simulink model "quat2mat"  (Simulink 6.1)
settings: Solver=ode45  StartTime=0.0  StopTime=10.0  RelTol=1e-3
libraries: simulink x1
settings Model: LastModifiedBy=okawa
settings DebuggingCC: SolverPrmCheckMsg=warning

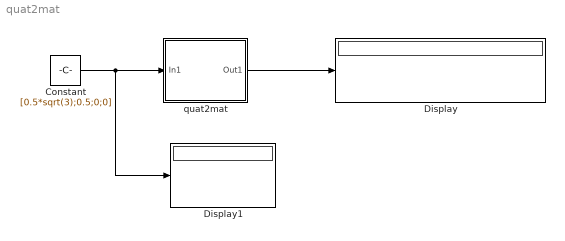
== system quat2mat ==
  Constant : Constant  Value=[0.5*sqrt(3);0.5;0;0]  VectorParams1D=off
  Display : Display
  Display1 : Display
  quat2mat : Subsystem
  wires:
  Constant/1 -> quat2mat/1(In1), Display1/1
  quat2mat/1(Out1) -> Display/1

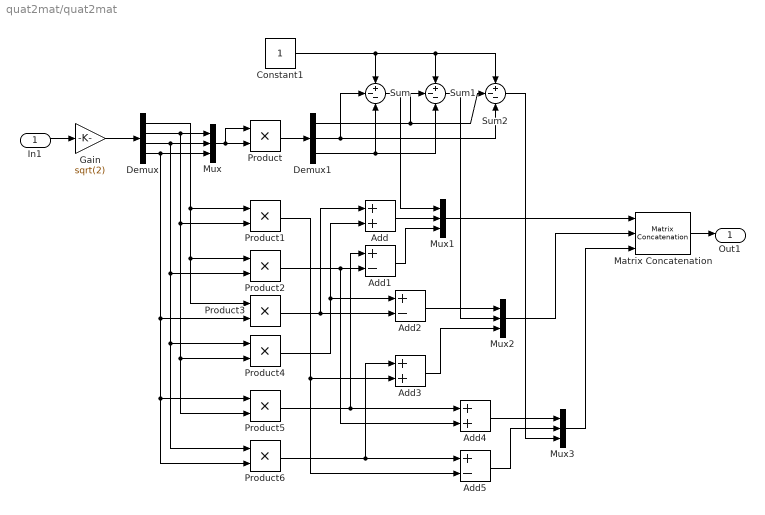
== system quat2mat/quat2mat ==
  In1 : Inport  Port=1  LatchInput=off
  Add : Sum  OutScaling=2^-10
  Add1 : Sum  Inputs=+-  OutScaling=2^-10
  Add2 : Sum  Inputs=+-  OutScaling=2^-10
  Add3 : Sum  OutScaling=2^-10
  Add4 : Sum  OutScaling=2^-10
  Add5 : Sum  Inputs=+-  OutScaling=2^-10
  Constant1 : Constant
  Demux : Demux
  Demux1 : Demux  Outputs=3
  Gain : Gain  Gain=sqrt(2)
  Matrix Concatenation : simulink/Math Operations/Matrix Concatenation  numInports=3  catMethod=Horizontal
  Mux{,1..3} (4 alike) : Mux  Inputs=3
  Product{,1..6} (7 alike) : Product  RndMeth=Zero
  Sum : Sum  Inputs=+--
  Sum1 : Sum  Inputs=+--
  Sum2 : Sum  Inputs=+--
  Out1 : Outport
  wires:
  Gain/1 -> Demux/1
  Demux/2 -> Mux/1, Product1/2, Product5/2, Product4/2
  Demux/3 -> Mux/2, Product6/1, Product4/1, Product2/2
  Demux/4 -> Mux/3, Product6/2, Product5/1, Product3/2
  Mux/1 -> Product/2, Product/1
  Product/1 -> Demux1/1
  Constant1/1 -> Sum/1, Sum2/1, Sum1/1
  Demux1/1 -> Sum2/2, Sum1/2
  Demux1/2 -> Sum2/3, Sum/2
  Demux1/3 -> Sum1/3, Sum/3
  Demux/1 -> Product1/1, Product3/1, Product2/1
  Mux1/1 -> Matrix Concatenation/1
  Mux3/1 -> Matrix Concatenation/3
  Mux2/1 -> Matrix Concatenation/2
  Add4/1 -> Mux3/1
  Add5/1 -> Mux3/2
  Sum2/1 -> Mux3/3
  Product6/1 -> Add5/1, Add3/1
  Product1/1 -> Add5/2, Add3/2
  Product5/1 -> Add4/1, Add1/1
  Add2/1 -> Mux2/1
  Sum1/1 -> Mux2/2
  Add3/1 -> Mux2/3
  Sum/1 -> Mux1/1
  Add/1 -> Mux1/2
  Add1/1 -> Mux1/3
  Product3/1 -> Add2/2, Add/1
  Product4/1 -> Add/2, Add2/1
  Product2/1 -> Add1/2, Add4/2
  In1/1 -> Gain/1
  Matrix Concatenation/1 -> Out1/1
